simulink model "Full_Hexacopter_Model"  (R2018a)
settings: Solver=VariableStepAuto  StartTime=0.0  StopTime=10.0  RelTol=1e-3
settings Model: Creator=Ibrahim  LastModifiedBy=Ibrahim

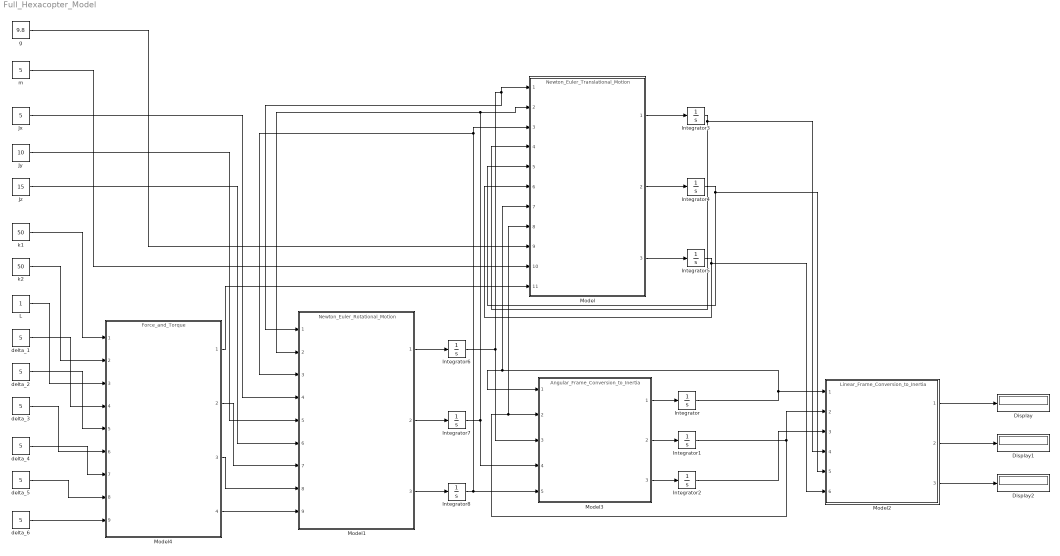
== system Full_Hexacopter_Model ==
  Display : Display
  Display1 : Display
  Display2 : Display
  Integrator{,1..8} (9 alike) : Integrator
  Jx : Constant  Value=5
  Jy : Constant  Value=10
  Jz : Constant  Value=15
  L : Constant
  Model : ModelReference  ModelNameDialog=Newton_Euler_Translational_Motion.slx  SimulationMode=Normal  ModelReferenceVersion=1.2
  Model1 : ModelReference  ModelNameDialog=Newton_Euler_Rotational_Motion.slx  SimulationMode=Normal  ModelReferenceVersion=1.1
  Model2 : ModelReference  ModelNameDialog=Linear_Frame_Conversion_to_Inertia.slx  SimulationMode=Normal  ModelReferenceVersion=1.8
  Model3 : ModelReference  ModelNameDialog=Angular_Frame_Conversion_to_Inertia.slx  SimulationMode=Normal  ModelReferenceVersion=1.10
  Model4 : ModelReference  ModelNameDialog=Force_and_Torque.slx  SimulationMode=Normal  ModelReferenceVersion=1.4
  delta_{1..6} (6 alike) : Constant  Value=5
  g : Constant  Value=9.8
  k1 : Constant  Value=50
  k2 : Constant  Value=50
  m : Constant  Value=5
  wires:
  Model4/4 -> Model1/9
  Model4/3 -> Model1/8
  Model4/2 -> Model1/7
  Model4/1 -> Model/11
  Model3/1 -> Integrator/1
  Model3/2 -> Integrator1/1
  Model3/3 -> Integrator2/1
  Integrator/1 -> Model/7, Model3/1, Model2/1
  Integrator1/1 -> Model2/2, Model/8, Model3/2
  Integrator2/1 -> Model2/3
  Model/2 -> Integrator4/1
  Model/1 -> Integrator3/1
  Model/3 -> Integrator5/1
  Integrator3/1 -> Model/4, Model2/4
  Integrator4/1 -> Model/5, Model2/5
  Integrator5/1 -> Model/6, Model2/6
  Model1/3 -> Integrator8/1
  Model1/2 -> Integrator7/1
  Model1/1 -> Integrator6/1
  Integrator6/1 -> Model1/1, Model/1, Model3/3
  Integrator7/1 -> Model1/2, Model/2, Model3/4
  Integrator8/1 -> Model1/3, Model/3, Model3/5
  g/1 -> Model/9
  m/1 -> Model/10
  delta_6/1 -> Model4/9
  delta_5/1 -> Model4/8
  delta_4/1 -> Model4/7
  delta_3/1 -> Model4/6
  delta_2/1 -> Model4/5
  delta_1/1 -> Model4/4
  L/1 -> Model4/3
  k2/1 -> Model4/2
  k1/1 -> Model4/1
  Jx/1 -> Model1/4
  Jy/1 -> Model1/5
  Jz/1 -> Model1/6
  Model2/1 -> Display/1
  Model2/2 -> Display1/1
  Model2/3 -> Display2/1
